simulink model "sampleModel653"  (R2023a)
settings: Solver=VariableStepAuto  StartTime=0.0  StopTime=10.0  RelTol=1e-3
undefined symbols (not defined in the file): DiscIntNeverNeededParam, magnitude, Newton, Raphson
libraries: simulink x238, slpidlib x68
(part 3 of 11)

== system sampleModel653/cfblk161 ==
  cfblk1 : Inport
  cfblk15 : Inport  Port=2
  cfblk10 : Product  Inputs=*
  cfblk11 : Signum
  cfblk12 : Constant  Value=[-980980330.453892]  SampleTime=1
  cfblk13 : Subsystem
  cfblk14 : Subsystem
  cfblk3 : DiscreteFir  SampleTime=1
  cfblk4 : slpidlib/PID Controller  Controller=PID  Form=Parallel  TimeDomain=Discrete-time  UseExternalTs=off  SampleTime=1  IntegratorMethod=Forward Euler  FilterMethod=Forward Euler  ControllerParametersSource=internal  P=1  I=1  UseKiTs=off  D=0  N=100  UseFilter=on  TunerSelectOption=Transfer Function Based (PID Tuner App)  InitialConditionSource=internal  InitialConditionForIntegrator=0  InitialConditionForFilter=0  DifferentiatorICPrevScaledInput=0  ExternalReset=none  TrackingMode=off  Kt=1  LimitOutput=off  SatLimitsSource=internal  UpperSaturationLimit=inf  LowerSaturationLimit=-inf  LinearizeAsGain=off  AntiWindupMode=none  Kb=1  LimitIntegrator=off  UpperIntegratorSaturationLimit=inf  LowerIntegratorSaturationLimit=-inf  POutMin=[]  POutMax=[]  IOutMin=[]  IOutMax=[]  DOutMin=[]  DOutMax=[]  NOutMin=[]  NOutMax=[]  SumOutMin=[]  SumOutMax=[]  SaturationOutMin=[]  SaturationOutMax=[]  PParamMin=[]  PParamMax=[]  IParamMin=[]  IParamMax=[]  DParamMin=[]  DParamMax=[]  NParamMin=[]  NParamMax=[]  KbParamMin=[]  KbParamMax=[]  KtParamMin=[]  KtParamMax=[]  KbOutMin=[]  KbOutMax=[]  KtOutMin=[]  KtOutMax=[]  IntegratorOutMin=[]  IntegratorOutMax=[]  FilterOutMin=[]  FilterOutMax=[]  SumI1OutMin=[]  SumI1OutMax=[]  SumI2OutMin=[]  SumI2OutMax=[]  SumI3OutMin=[]  SumI3OutMax=[]  SumI4OutMin=[]  SumI4OutMax=[]  SumDOutMin=[]  SumDOutMax=[]  DifferentiatorOutMin=[]  DifferentiatorOutMax=[]  FilterDiffOutCoefMin=[]  FilterDiffOutCoefMax=[]  ReciprocalOutMin=[]  ReciprocalOutMax=[]  SumDenOutMin=[]  SumDenOutMax=[]  SumNumOutMin=[]  SumNumOutMax=[]  DivideOutMin=[]  DivideOutMax=[]  UdiffTsProdOutMin=[]  UdiffTsProdOutMax=[]  NTsProdOutMin=[]  NTsProdOutMax=[]  UintegralTsProdOutMin=[]  UintegralTsProdOutMax=[]  UngainTsProdOutMin=[]  UngainTsProdOutMax=[]  ClampingZeroOutDataTypeStr=Inherit: Inherit via back propagation  ClampingZeroOutMin=[]  ClampingZeroOutMax=[]  FilterDenConstantOutDataTypeStr=Inherit: Inherit via back propagation  FilterDenConstantOutMin=[]  FilterDenConstantOutMax=[]  PCopyOutDataTypeStr=Inherit: Inherit via back propagation  PCopyOutMin=[]  PCopyOutMax=[]  NCopyOutDataTypeStr=Inherit: Inherit via back propagation  NCopyOutMin=[]  NCopyOutMax=[]  IntegratorContinuousStateAttributes=''  IntegratorStateMustResolveToSignalObject=off  IntegratorRTWStateStorageClass=Auto  FilterContinuousStateAttributes=''  FilterStateMustResolveToSignalObject=off  FilterRTWStateStorageClass=Auto  ParallelPVariant=InternalParameters  IdealPVariant=Disabled  IVariant=InternalParameters  DVariant=InternalParameters  IntegratorVariant=Discrete  SatVariant=Disabled  AWVariant=Passthrough  PCopyVariant=Disabled  TRVariant=Disabled  FdbkBlocksVariant=Forward  IdealPFdbkVariant=Disabled  SatFdbkVariant=Disabled  DerivativeFilterVariant=ForwardEulerFilter  NVariant=InternalParameters  NCopyVariant=Disabled  FilterICVariant=InternalICsFilter  IntegratorICVariant=InternalICs  ExternalResetVariant=Disabled  TRSumVariant=Passthrough  SumFdbkVariant=Disabled  SumVariant=Sum_PID  TsampFilterVariant=InternalTs  TsampNgainVariant=Passthrough  TsampIntegralVariant=Disabled_SignalSpec  ExternalSaturationOutDataTypeStr=Inherit: Same as second input
      settings: LibrarySourceBlock=simulink/Discrete/Discrete PID Controller
  cfblk5 : simulink/Discrete/Tapped Delay  vinit=0.0  samptime=-1  NumDelays=1  DelayOrder=Oldest  includeCurrent=off
  cfblk6 : Sum  Inputs=+-
  cfblk7 : Sqrt  Operator=rSqrt  AlgorithmType=Newton-Raphson
  cfblk8 : ComplexToMagnitudeAngle
  cfblk9 : Math  Operator=conj
  cfblk2 : Outport
  cfblk16 : Outport  Port=2
  wires:
  cfblk7/1 -> cfblk6/1
  cfblk14/1(cfblk2) -> cfblk16/1
  cfblk4/1 -> cfblk7/1
  cfblk6/1 -> cfblk14/1(cfblk1)
  cfblk12/1 -> cfblk8/1
  cfblk5/1 -> cfblk3/1
  cfblk9/1 -> cfblk14/2(cfblk6)
  cfblk14/2(cfblk7) -> cfblk10/1
  cfblk8/1 -> cfblk13/1(cfblk1)
  cfblk11/1 -> cfblk9/1
  cfblk15/1 -> cfblk13/2(cfblk13)
  cfblk13/1(cfblk2) -> cfblk6/2
  cfblk3/1 -> cfblk11/1
  cfblk8/2 -> cfblk5/1
  cfblk1/1 -> cfblk4/1
  cfblk13/2(cfblk14) -> cfblk2/1

== system sampleModel653/cfblk162 ==
  cfblk1 : Inport
  cfblk12 : Inport  Port=2
  cfblk13 : Inport  Port=3
  cfblk10 : Subsystem
  cfblk11 : Subsystem
  cfblk{14..17} (4 alike) : Delay  SampleTime=1
  cfblk3 : DiscreteStateSpace
  cfblk4 : simulink/Discrete/Difference  ICPrevInput=0.0  OutMin=[]  OutMax=[]  OutDataTypeStr=Inherit: Inherit via back propagation  OutDataType=fixdt(1, 16)  OutScaling=2^-10  DoSatur=off
  cfblk5 : simulink/Math Operations/Slider Gain  gain=1  low=0  high=2
  cfblk6 : Constant  Value=[520175118.847809]  SampleTime=1
  cfblk7 : Subsystem
  cfblk8 : Subsystem
  cfblk9 : Subsystem
  cfblk2 : Outport
  wires:
  cfblk7/1(cfblk2) -> cfblk4/1
  cfblk12/1 -> cfblk11/1(cfblk1)
  cfblk11/1(cfblk2) -> cfblk3/1
  cfblk13/1 -> cfblk7/1(cfblk1)
  cfblk6/1 -> cfblk11/3(cfblk15), cfblk10/2(cfblk6)
  cfblk1/1 -> cfblk11/4(cfblk16)
  cfblk5/1 -> cfblk8/2(cfblk7)
  cfblk7/2(cfblk15) -> cfblk5/1
  cfblk8/2(cfblk9) -> cfblk9/1(cfblk1)
  cfblk10/1(cfblk2) -> cfblk2/1
  cfblk8/3(cfblk10) -> cfblk9/2(cfblk14)
  cfblk3/1 -> cfblk7/3(cfblk14)
  cfblk7/3(cfblk16) -> cfblk9/3(cfblk15)
  cfblk9/3(cfblk17) -> cfblk10/1(cfblk1)
  cfblk4/1 -> cfblk14/1
  cfblk14/1 -> cfblk11/2(cfblk14)
  cfblk8/1(cfblk2) -> cfblk15/1
  cfblk15/1 -> cfblk7/2(cfblk13)
  cfblk9/1(cfblk2) -> cfblk16/1
  cfblk16/1 -> cfblk8/1(cfblk1)
  cfblk9/2(cfblk16) -> cfblk17/1
  cfblk17/1 -> cfblk8/3(cfblk8)

== system sampleModel653/cfblk163 ==
  cfblk1 : Inport
  cfblk3 : simulink/Discrete/Transfer Fcn First Order  PoleZ=0.95  ICPrevOutput=0.0  DoSatur=off
  cfblk4 : Product  Inputs=**
  cfblk5 : Sum  Inputs=--
  cfblk6 : Abs  SaturateOnIntegerOverflow=off
  cfblk7 : Constant  Value=[266211671.237557]  SampleTime=1
  cfblk2 : Outport
  cfblk8 : Outport  Port=2
  cfblk9 : Outport  Port=3
  wires:
  cfblk1/1 -> cfblk6/1
  cfblk3/1 -> cfblk5/1
  cfblk4/1 -> cfblk9/1
  cfblk6/1 -> cfblk5/2, cfblk3/1
  cfblk5/1 -> cfblk4/1, cfblk8/1
  cfblk7/1 -> cfblk2/1, cfblk4/2

== system sampleModel653/cfblk164 ==
  cfblk1 : Inport
  cfblk7 : Inport  Port=2
  cfblk8 : Inport  Port=3
  cfblk3 : simulink/Discrete/Transfer Fcn First Order  PoleZ=0.95  ICPrevOutput=0.0  DoSatur=off
  cfblk4 : simulink/Discrete/Transfer Fcn Real Zero  ZeroZ=0.75  ICPrevInput=0.0  DoSatur=off
  cfblk5 : Constant  Value=[908519091.701283]  SampleTime=1
  cfblk6 : Subsystem
  cfblk9 : Delay  SampleTime=1
  cfblk2 : Outport
  wires:
  cfblk1/1 -> cfblk2/1, cfblk6/5(cfblk15)
  cfblk5/1 -> cfblk6/1(cfblk1)
  cfblk4/1 -> cfblk6/2(cfblk12)
  cfblk6/1(cfblk2) -> cfblk3/1
  cfblk8/1 -> cfblk6/4(cfblk14)
  cfblk7/1 -> cfblk4/1
  cfblk3/1 -> cfblk9/1
  cfblk9/1 -> cfblk6/3(cfblk13)

== system sampleModel653/cfblk165 ==
  cfblk1 : Inport
  cfblk8 : Inport  Port=2
  cfblk9 : Inport  Port=3
  cfblk3 : simulink/Discrete/Tapped Delay  vinit=0.0  samptime=-1  NumDelays=1  DelayOrder=Oldest  includeCurrent=off
  cfblk4 : UnitDelay  HasFrameUpgradeWarning=on
  cfblk5 : Sqrt
  cfblk6 : ComplexToMagnitudeAngle
  cfblk7 : Subsystem
  cfblk2 : Outport
  cfblk10 : Outport  Port=2
  wires:
  cfblk4/1 -> cfblk10/1
  cfblk5/1 -> cfblk7/1(cfblk1)
  cfblk3/1 -> cfblk6/1
  cfblk6/1 -> cfblk4/1
  cfblk7/1(cfblk2) -> cfblk3/1
  cfblk1/1 -> cfblk5/1
  cfblk7/2(cfblk6) -> cfblk2/1

== system sampleModel653/cfblk166 ==
  cfblk1 : Inport
  cfblk{4,11..15} (6 alike) : Delay  SampleTime=1
  cfblk3 : Delay  DelayLengthSource=Input port  SampleTime=1
      settings: InputPortMap=u0,p1
  cfblk5 : Sqrt  Operator=rSqrt  AlgorithmType=Newton-Raphson
  cfblk6 : Product  Inputs=*
  cfblk7 : Subsystem
  cfblk2 : Outport
  cfblk8 : Outport  Port=2
  cfblk9 : Outport  Port=3
  cfblk10 : Outport  Port=4
  wires:
  cfblk4/1 -> cfblk8/1, cfblk12/1, cfblk13/1
  cfblk3/1 -> cfblk4/1, cfblk2/1, cfblk11/1, cfblk14/1
  cfblk1/1 -> cfblk6/1, cfblk7/5(cfblk13), cfblk7/6(cfblk14)
  cfblk7/1(cfblk2) -> cfblk5/1, cfblk9/1
  cfblk6/1 -> cfblk10/1, cfblk7/3(cfblk11)
  cfblk5/1 -> cfblk3/2, cfblk15/1
  cfblk11/1 -> cfblk7/1(cfblk1)
  cfblk12/1 -> cfblk3/1
  cfblk13/1 -> cfblk7/4(cfblk12)
  cfblk14/1 -> cfblk7/2(cfblk10)
  cfblk15/1 -> cfblk7/7(cfblk15)

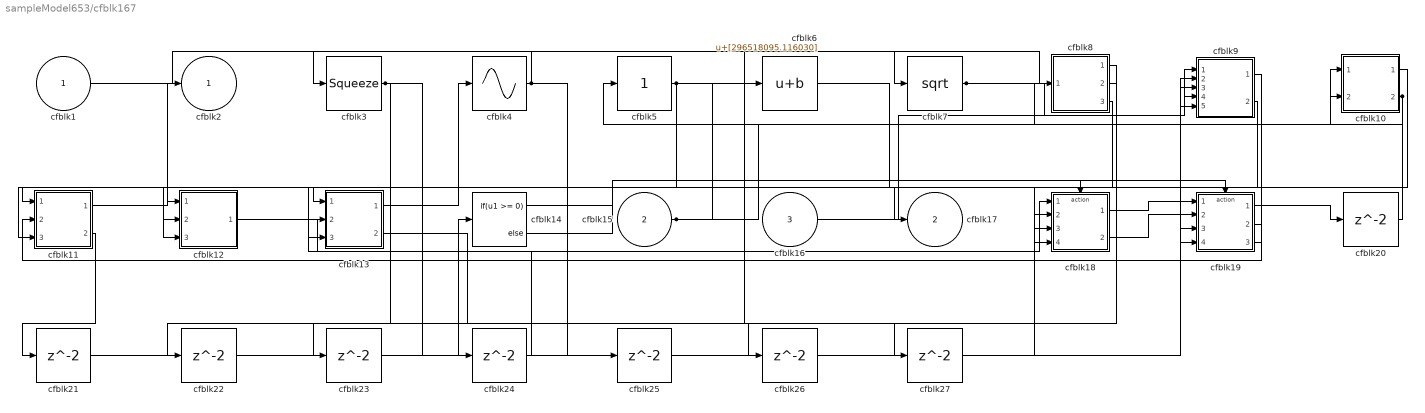
== system sampleModel653/cfblk167 ==
  cfblk1 : Inport
  cfblk15 : Inport  Port=2
  cfblk16 : Inport  Port=3
  cfblk10 : Subsystem
  cfblk11 : Subsystem
  cfblk12 : Subsystem
  cfblk13 : Subsystem
  cfblk14 : If  IfExpression=u1 >= 0  SampleTime=1
  cfblk18 : Subsystem  TreatAsAtomicUnit=on
  cfblk19 : Subsystem  TreatAsAtomicUnit=on
  cfblk{20..27} (8 alike) : Delay  SampleTime=1
  cfblk3 : Squeeze
  cfblk4 : Sin  TimeSource=Use external signal  SampleTime=0
  cfblk5 : simulink/Math Operations/Slider Gain  gain=1  low=0  high=2
  cfblk6 : Bias  Bias=[296518095.116030]  SaturateOnIntegerOverflow=off
  cfblk7 : Sqrt
  cfblk8 : Subsystem
  cfblk9 : Subsystem
  cfblk2 : Outport
  cfblk17 : Outport  Port=2
  wires:
  cfblk16/1 -> cfblk9/1(cfblk1)
  cfblk5/1 -> cfblk11/1(cfblk1), cfblk8/1(cfblk1), cfblk13/3(cfblk16), cfblk27/1
  cfblk13/1(cfblk2) -> cfblk4/1
  cfblk12/1(cfblk2) -> cfblk18/1(cfblk1)
  cfblk15/1 -> cfblk6/1, cfblk10/1(cfblk1)
  cfblk1/1 -> cfblk7/1
  cfblk11/1(cfblk2) -> cfblk2/1
  cfblk9/1(cfblk2) -> cfblk12/1(cfblk1)
  cfblk19/2(cfblk16) -> cfblk11/2(cfblk14)
  cfblk4/1 -> cfblk3/1, cfblk25/1
  cfblk19/3(cfblk17) -> cfblk5/1
  cfblk3/1 -> cfblk23/1, cfblk24/1
  cfblk6/1 -> cfblk18/4(cfblk12)
  cfblk9/2(cfblk15) -> cfblk12/2(cfblk10)
  cfblk10/1(cfblk2) -> cfblk13/1(cfblk1)
  cfblk8/1(cfblk2) -> cfblk17/1
  cfblk10/2(cfblk10) -> cfblk12/3(cfblk11), cfblk19/4(cfblk15)
  cfblk18/1(cfblk2) -> cfblk19/1(cfblk1)
  cfblk18/2(cfblk13) -> cfblk19/2(cfblk13)
  cfblk7/1 -> cfblk9/4(cfblk13), cfblk10/2(cfblk9)
  cfblk8/3(cfblk8) -> cfblk11/3(cfblk15)
  cfblk14/1 -> cfblk18/Action
  cfblk14/2 -> cfblk19/Action
  cfblk19/1(cfblk2) -> cfblk20/1
  cfblk20/1 -> cfblk9/2(cfblk11)
  cfblk11/2(cfblk16) -> cfblk21/1
  cfblk21/1 -> cfblk18/3(cfblk11)
  cfblk8/2(cfblk7) -> cfblk22/1
  cfblk22/1 -> cfblk14/1
  cfblk23/1 -> cfblk9/3(cfblk12)
  cfblk24/1 -> cfblk13/2(cfblk15)
  cfblk25/1 -> cfblk19/3(cfblk14)
  cfblk13/2(cfblk17) -> cfblk26/1
  cfblk26/1 -> cfblk18/2(cfblk10)
  cfblk27/1 -> cfblk9/5(cfblk14)

== system sampleModel653/cfblk168 ==
  cfblk1 : Inport
  cfblk10 : Inport  Port=2
  cfblk11 : Inport  Port=3
  cfblk13 : Delay  SampleTime=1
  cfblk3 : DiscreteStateSpace
  cfblk4 : DiscreteZeroPole  Poles=[0 0.5]  Gain=1
  cfblk5 : Rounding
  cfblk6 : Constant  Value=[-270536108.495275]  SampleTime=1
  cfblk7 : Subsystem
  cfblk8 : Subsystem
  cfblk9 : Subsystem
  cfblk2 : Outport
  cfblk12 : Outport  Port=2
  wires:
  cfblk1/1 -> cfblk7/1(cfblk1)
  cfblk11/1 -> cfblk8/1(cfblk1)
  cfblk6/1 -> cfblk8/2(cfblk10)
  cfblk3/1 -> cfblk2/1
  cfblk9/1(cfblk2) -> cfblk12/1
  cfblk4/1 -> cfblk9/1(cfblk1)
  cfblk8/1(cfblk2) -> cfblk3/1
  cfblk10/1 -> cfblk5/1
  cfblk8/2(cfblk11) -> cfblk9/2(cfblk8)
  cfblk9/2(cfblk9) -> cfblk13/1
  cfblk13/1 -> cfblk4/1

== system sampleModel653/cfblk169 ==
  cfblk1 : Inport
  cfblk7 : Inport  Port=2
  cfblk3 : Constant  Value=[373927512.445673]  SampleTime=1
  cfblk4 : Constant  Value=[-436487022.604392]  SampleTime=1
  cfblk5 : Subsystem
  cfblk6 : Subsystem
  cfblk8 : Delay  SampleTime=1
  cfblk2 : Outport
  wires:
  cfblk1/1 -> cfblk2/1
  cfblk6/1(cfblk2) -> cfblk5/1(cfblk1)
  cfblk7/1 -> cfblk6/1(cfblk1)
  cfblk4/1 -> cfblk6/3(cfblk10)
  cfblk5/1(cfblk2) -> cfblk8/1
  cfblk8/1 -> cfblk6/2(cfblk9)

== system sampleModel653/cfblk170 ==
  cfblk1 : Inport
  cfblk13 : Inport  Port=2
  cfblk14 : Inport  Port=3
  cfblk10 : Subsystem
  cfblk11 : Subsystem
  cfblk12 : Subsystem
  cfblk15 : Delay  SampleTime=1
  cfblk16 : Delay  SampleTime=1
  cfblk3 : Sum  Inputs=+-
  cfblk4 : UnaryMinus
  cfblk5 : Sum  Inputs=+-
  cfblk6 : Rounding
  cfblk7 : simulink/Math Operations/Slider Gain  gain=1  low=0  high=2
  cfblk8 : Sum  Inputs=+-
  cfblk9 : Constant  Value=[279332915.374205]  SampleTime=1
  cfblk2 : Outport
  wires:
  cfblk13/1 -> cfblk6/1, cfblk10/4(cfblk15)
  cfblk1/1 -> cfblk3/1
  cfblk6/1 -> cfblk7/1, cfblk10/3(cfblk14)
  cfblk9/1 -> cfblk10/1(cfblk1), cfblk11/3(cfblk15)
  cfblk11/1(cfblk2) -> cfblk5/1
  cfblk4/1 -> cfblk11/1(cfblk1), cfblk11/4(cfblk16)
  cfblk14/1 -> cfblk5/2
  cfblk7/1 -> cfblk4/1
  cfblk10/1(cfblk2) -> cfblk12/1(cfblk1)
  cfblk12/1(cfblk2) -> cfblk8/1
  cfblk5/1 -> cfblk8/2
  cfblk11/2(cfblk17) -> cfblk2/1
  cfblk3/1 -> cfblk11/2(cfblk14)
  cfblk8/1 -> cfblk15/1
  cfblk15/1 -> cfblk3/2
  cfblk12/2(cfblk8) -> cfblk16/1
  cfblk16/1 -> cfblk10/2(cfblk13)

== system sampleModel653/cfblk171 ==
  cfblk1 : Inport
  cfblk8 : Inport  Port=2
  cfblk9 : Inport  Port=3
  cfblk11 : Delay  SampleTime=1
  cfblk3 : slpidlib/PID Controller (2DOF)  Controller=PID  Form=Parallel  TimeDomain=Discrete-time  UseExternalTs=off  SampleTime=1  IntegratorMethod=Forward Euler  FilterMethod=Forward Euler  ControllerParametersSource=internal  P=1  I=1  UseKiTs=off  D=0  N=100  UseFilter=on  b=1  c=1  TunerSelectOption=Transfer Function Based (PID Tuner App)  InitialConditionSource=internal  InitialConditionForIntegrator=0  InitialConditionForFilter=0  DifferentiatorICPrevScaledInput=0  ExternalReset=none  TrackingMode=off  Kt=1  LimitOutput=off  SatLimitsSource=internal  UpperSaturationLimit=inf  LowerSaturationLimit=-inf  LinearizeAsGain=off  AntiWindupMode=none  Kb=1  LimitIntegrator=off  UpperIntegratorSaturationLimit=inf  LowerIntegratorSaturationLimit=-inf  POutMin=[]  POutMax=[]  IOutMin=[]  IOutMax=[]  DOutMin=[]  DOutMax=[]  NOutMin=[]  NOutMax=[]  bOutMin=[]  bOutMax=[]  cOutMin=[]  cOutMax=[]  SumOutMin=[]  SumOutMax=[]  SaturationOutMin=[]  SaturationOutMax=[]  PParamMin=[]  PParamMax=[]  IParamMin=[]  IParamMax=[]  DParamMin=[]  DParamMax=[]  NParamMin=[]  NParamMax=[]  bParamMin=[]  bParamMax=[]  cParamMin=[]  cParamMax=[]  KbParamMin=[]  KbParamMax=[]  KtParamMin=[]  KtParamMax=[]  KbOutMin=[]  KbOutMax=[]  KtOutMin=[]  KtOutMax=[]  IntegratorOutMin=[]  IntegratorOutMax=[]  FilterOutMin=[]  FilterOutMax=[]  SumI1OutMin=[]  SumI1OutMax=[]  SumI2OutMin=[]  SumI2OutMax=[]  SumI3OutMin=[]  SumI3OutMax=[]  SumI4OutMin=[]  SumI4OutMax=[]  SumDOutMin=[]  SumDOutMax=[]  Sum1OutMin=[]  Sum1OutMax=[]  Sum2OutMin=[]  Sum2OutMax=[]  Sum3OutMin=[]  Sum3OutMax=[]  DifferentiatorOutMin=[]  DifferentiatorOutMax=[]  FilterDiffOutCoefMin=[]  FilterDiffOutCoefMax=[]  ReciprocalOutMin=[]  ReciprocalOutMax=[]  SumDenOutMin=[]  SumDenOutMax=[]  SumNumOutMin=[]  SumNumOutMax=[]  DivideOutMin=[]  DivideOutMax=[]  UdiffTsProdOutMin=[]  UdiffTsProdOutMax=[]  NTsProdOutMin=[]  NTsProdOutMax=[]  UintegralTsProdOutMin=[]  UintegralTsProdOutMax=[]  UngainTsProdOutMin=[]  UngainTsProdOutMax=[]  ClampingZeroOutDataTypeStr=Inherit: Inherit via back propagation  ClampingZeroOutMin=[]  ClampingZeroOutMax=[]  FilterDenConstantOutDataTypeStr=Inherit: Inherit via back propagation  FilterDenConstantOutMin=[]  FilterDenConstantOutMax=[]  PCopyOutDataTypeStr=Inherit: Inherit via back propagation  PCopyOutMin=[]  PCopyOutMax=[]  NCopyOutDataTypeStr=Inherit: Inherit via back propagation  NCopyOutMin=[]  NCopyOutMax=[]  IntegratorContinuousStateAttributes=''  IntegratorStateMustResolveToSignalObject=off  IntegratorRTWStateStorageClass=Auto  FilterContinuousStateAttributes=''  FilterStateMustResolveToSignalObject=off  FilterRTWStateStorageClass=Auto  ParallelPVariant=InternalParameters  IdealPVariant=Disabled  IVariant=InternalParameters  DVariant=InternalParameters  bVariant=InternalParameters  cVariant=InternalParameters  IntegratorVariant=Discrete  SatVariant=Disabled  AWVariant=Passthrough  PCopyVariant=Disabled  TRVariant=Disabled  FdbkBlocksVariant=Forward  IdealPFdbkVariant=Disabled  SatFdbkVariant=Disabled  DerivativeFilterVariant=ForwardEulerFilter  NVariant=InternalParameters  NCopyVariant=Disabled  FilterICVariant=InternalICsFilter  IntegratorICVariant=InternalICs  ExternalResetVariant=Disabled  TRSumVariant=Passthrough  SumFdbkVariant=Disabled  SumVariant=Sum_PID  TsampFilterVariant=InternalTs  TsampNgainVariant=Passthrough  TsampIntegralVariant=Disabled_SignalSpec  ExternalSaturationOutDataTypeStr=Inherit: Same as second input
      settings: LibrarySourceBlock=simulink/Discrete/Discrete PID Controller (2DOF)
  cfblk4 : Gain  Gain=[-457446233.510132]
  cfblk5 : Constant  Value=[-436711553.418226]  SampleTime=1
  cfblk6 : Subsystem
  cfblk7 : Subsystem
  cfblk2 : Outport
  cfblk10 : Outport  Port=2
  wires:
  cfblk7/1(cfblk2) -> cfblk10/1
  cfblk5/1 -> cfblk2/1
  cfblk4/1 -> cfblk6/1(cfblk1), cfblk7/3(cfblk7)
  cfblk1/1 -> cfblk7/1(cfblk1)
  cfblk8/1 -> cfblk6/2(cfblk15), cfblk3/2
  cfblk9/1 -> cfblk6/3(cfblk16)
  cfblk6/1(cfblk2) -> cfblk7/2(cfblk6), cfblk11/1
  cfblk3/1 -> cfblk4/1
  cfblk11/1 -> cfblk3/1

== system sampleModel653/cfblk172 ==
  cfblk1 : Inport
  cfblk6 : Inport  Port=2
  cfblk{10..13} (4 alike) : Delay  SampleTime=1
  cfblk3 : Delay  ShowEnablePort=on  SampleTime=1
      settings: InputPortMap=u0,e6
  cfblk4 : Sum  Inputs=--
  cfblk5 : Subsystem
  cfblk2 : Outport
  cfblk7 : Outport  Port=2
  cfblk8 : Outport  Port=3
  cfblk9 : Outport  Port=4
  wires:
  cfblk4/1 -> cfblk8/1, cfblk5/5(cfblk12)
  cfblk6/1 -> cfblk3/1, cfblk9/1
  cfblk5/1(cfblk2) -> cfblk3/2
  cfblk1/1 -> cfblk4/2, cfblk5/2(cfblk9)
  cfblk3/1 -> cfblk2/1, cfblk7/1, cfblk10/1, cfblk11/1, cfblk12/1
  cfblk10/1 -> cfblk5/1(cfblk1)
  cfblk11/1 -> cfblk5/3(cfblk10)
  cfblk12/1 -> cfblk5/4(cfblk11)
  cfblk5/2(cfblk13) -> cfblk13/1
  cfblk13/1 -> cfblk4/1

== system sampleModel653/cfblk173 ==
  cfblk1 : Inport
  cfblk7 : Inport  Port=2
  cfblk3 : Delay  DelayLengthSource=Input port  SampleTime=1
      settings: InputPortMap=u0,p1
  cfblk4 : DiscreteZeroPole  Poles=[0 0.5]  Gain=1
  cfblk5 : Signum
  cfblk6 : Subsystem
  cfblk8 : Delay  SampleTime=1
  cfblk2 : Outport
  wires:
  cfblk6/1(cfblk2) -> cfblk4/1
  cfblk4/1 -> cfblk2/1
  cfblk6/2(cfblk9) -> cfblk3/1
  cfblk5/1 -> cfblk3/2
  cfblk7/1 -> cfblk5/1
  cfblk1/1 -> cfblk6/1(cfblk1)
  cfblk3/1 -> cfblk8/1
  cfblk8/1 -> cfblk6/2(cfblk8)

== system sampleModel653/cfblk183 ==
  cfblk1 : Inport
  cfblk8 : Inport  Port=2
  Action Port : ActionPort  ActionPortLabel=if(u1 >= 0)
  cfblk3 : Squeeze
  cfblk4 : Reshape
  cfblk5 : Constant  Value=[-334139740.220997]  SampleTime=1
  cfblk6 : Constant  Value=[-428556013.443740]  SampleTime=1
  cfblk7 : Subsystem
  cfblk2 : Outport
  wires:
  cfblk5/1 -> cfblk2/1
  cfblk6/1 -> cfblk4/1
  cfblk1/1 -> cfblk3/1
  cfblk4/1 -> cfblk7/1(cfblk1)
  cfblk8/1 -> cfblk7/2(cfblk15)
  cfblk3/1 -> cfblk7/3(cfblk16)

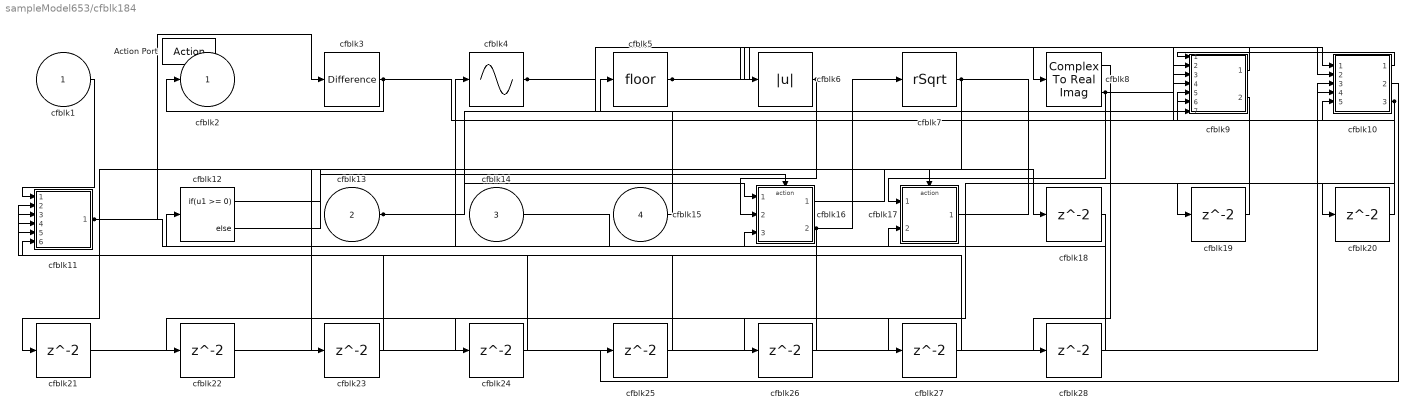
== system sampleModel653/cfblk184 ==
  cfblk1 : Inport
  cfblk13 : Inport  Port=2
  cfblk14 : Inport  Port=3
  cfblk15 : Inport  Port=4
  Action Port : ActionPort  ActionPortLabel=else
  cfblk10 : Subsystem
  cfblk11 : Subsystem
  cfblk12 : If  IfExpression=u1 >= 0  SampleTime=1
  cfblk16 : Subsystem  TreatAsAtomicUnit=on
  cfblk17 : Subsystem  TreatAsAtomicUnit=on
  cfblk{18..28} (11 alike) : Delay
  cfblk3 : simulink/Discrete/Difference  ICPrevInput=0.0  OutMin=[]  OutMax=[]  OutDataTypeStr=Inherit: Inherit via back propagation  OutDataType=fixdt(1, 16)  OutScaling=2^-10  DoSatur=off
  cfblk4 : Sin  TimeSource=Use external signal  SampleTime=0
  cfblk5 : Rounding
  cfblk6 : Abs  SaturateOnIntegerOverflow=off
  cfblk7 : Sqrt  Operator=rSqrt  AlgorithmType=Newton-Raphson
  cfblk8 : ComplexToRealImag
  cfblk9 : Subsystem
  cfblk2 : Outport
  wires:
  cfblk13/1 -> cfblk16/1(cfblk1), cfblk9/5(cfblk13)
  cfblk10/1(cfblk2) -> cfblk9/1(cfblk1)
  cfblk3/1 -> cfblk2/1, cfblk10/5(cfblk14)
  cfblk16/2(cfblk16) -> cfblk7/1, cfblk22/1
  cfblk6/1 -> cfblk16/2(cfblk14), cfblk23/1
  cfblk14/1 -> cfblk16/3(cfblk15)
  cfblk5/1 -> cfblk9/3(cfblk11), cfblk10/1(cfblk1)
  cfblk15/1 -> cfblk5/1
  cfblk11/1(cfblk2) -> cfblk3/1, cfblk17/2(cfblk8)
  cfblk9/1(cfblk2) -> cfblk6/1
  cfblk4/1 -> cfblk8/1, cfblk9/6(cfblk14)
  cfblk1/1 -> cfblk11/1(cfblk1)
  cfblk7/1 -> cfblk20/1, cfblk21/1
  cfblk8/2 -> cfblk17/1(cfblk1), cfblk10/2(cfblk11)
  cfblk10/3(cfblk16) -> cfblk9/7(cfblk15), cfblk26/1, cfblk27/1
  cfblk12/1 -> cfblk16/Action
  cfblk12/2 -> cfblk17/Action
  cfblk16/1(cfblk2) -> cfblk18/1
  cfblk18/1 -> cfblk12/1
  cfblk17/1(cfblk2) -> cfblk19/1
  cfblk19/1 -> cfblk9/2(cfblk10)
  cfblk20/1 -> cfblk9/4(cfblk12)
  cfblk21/1 -> cfblk10/3(cfblk12)
  cfblk22/1 -> cfblk10/4(cfblk13)
  cfblk23/1 -> cfblk11/5(cfblk14)
  cfblk9/2(cfblk16) -> cfblk24/1
  cfblk24/1 -> cfblk11/2(cfblk11)
  cfblk10/2(cfblk15) -> cfblk25/1
  cfblk25/1 -> cfblk11/3(cfblk12)
  cfblk26/1 -> cfblk11/4(cfblk13)
  cfblk27/1 -> cfblk11/6(cfblk15)
  cfblk8/1 -> cfblk28/1
  cfblk28/1 -> cfblk4/1

== system sampleModel653/cfblk185 ==
  cfblk1 : Inport
  Action Port : ActionPort  ActionPortLabel=if(u1 >= 0)
  cfblk10 : Constant  Value=[724663783.826056]  SampleTime=1
  cfblk11 : Subsystem
  cfblk12 : Subsystem
  cfblk3 : simulink/Discrete/Transfer Fcn First Order  PoleZ=0.95  ICPrevOutput=0.0  DoSatur=off
  cfblk4 : slpidlib/PID Controller  Controller=PID  Form=Parallel  TimeDomain=Discrete-time  UseExternalTs=off  SampleTime=-1  IntegratorMethod=Forward Euler  FilterMethod=Forward Euler  ControllerParametersSource=internal  P=1  I=1  UseKiTs=off  D=0  N=100  UseFilter=on  TunerSelectOption=Transfer Function Based (PID Tuner App)  InitialConditionSource=internal  InitialConditionForIntegrator=0  InitialConditionForFilter=0  DifferentiatorICPrevScaledInput=0  ExternalReset=none  TrackingMode=off  Kt=1  LimitOutput=off  SatLimitsSource=internal  UpperSaturationLimit=inf  LowerSaturationLimit=-inf  LinearizeAsGain=off  AntiWindupMode=none  Kb=1  LimitIntegrator=off  UpperIntegratorSaturationLimit=inf  LowerIntegratorSaturationLimit=-inf  POutMin=[]  POutMax=[]  IOutMin=[]  IOutMax=[]  DOutMin=[]  DOutMax=[]  NOutMin=[]  NOutMax=[]  SumOutMin=[]  SumOutMax=[]  SaturationOutMin=[]  SaturationOutMax=[]  PParamMin=[]  PParamMax=[]  IParamMin=[]  IParamMax=[]  DParamMin=[]  DParamMax=[]  NParamMin=[]  NParamMax=[]  KbParamMin=[]  KbParamMax=[]  KtParamMin=[]  KtParamMax=[]  KbOutMin=[]  KbOutMax=[]  KtOutMin=[]  KtOutMax=[]  IntegratorOutMin=[]  IntegratorOutMax=[]  FilterOutMin=[]  FilterOutMax=[]  SumI1OutMin=[]  SumI1OutMax=[]  SumI2OutMin=[]  SumI2OutMax=[]  SumI3OutMin=[]  SumI3OutMax=[]  SumI4OutMin=[]  SumI4OutMax=[]  SumDOutMin=[]  SumDOutMax=[]  DifferentiatorOutMin=[]  DifferentiatorOutMax=[]  FilterDiffOutCoefMin=[]  FilterDiffOutCoefMax=[]  ReciprocalOutMin=[]  ReciprocalOutMax=[]  SumDenOutMin=[]  SumDenOutMax=[]  SumNumOutMin=[]  SumNumOutMax=[]  DivideOutMin=[]  DivideOutMax=[]  UdiffTsProdOutMin=[]  UdiffTsProdOutMax=[]  NTsProdOutMin=[]  NTsProdOutMax=[]  UintegralTsProdOutMin=[]  UintegralTsProdOutMax=[]  UngainTsProdOutMin=[]  UngainTsProdOutMax=[]  ClampingZeroOutDataTypeStr=Inherit: Inherit via back propagation  ClampingZeroOutMin=[]  ClampingZeroOutMax=[]  FilterDenConstantOutDataTypeStr=Inherit: Inherit via back propagation  FilterDenConstantOutMin=[]  FilterDenConstantOutMax=[]  PCopyOutDataTypeStr=Inherit: Inherit via back propagation  PCopyOutMin=[]  PCopyOutMax=[]  NCopyOutDataTypeStr=Inherit: Inherit via back propagation  NCopyOutMin=[]  NCopyOutMax=[]  IntegratorContinuousStateAttributes=''  IntegratorStateMustResolveToSignalObject=off  IntegratorRTWStateStorageClass=Auto  FilterContinuousStateAttributes=''  FilterStateMustResolveToSignalObject=off  FilterRTWStateStorageClass=Auto  ParallelPVariant=InternalParameters  IdealPVariant=Disabled  IVariant=InternalParameters  DVariant=InternalParameters  IntegratorVariant=Discrete  SatVariant=Disabled  AWVariant=Passthrough  PCopyVariant=Disabled  TRVariant=Disabled  FdbkBlocksVariant=Forward  IdealPFdbkVariant=Disabled  SatFdbkVariant=Disabled  DerivativeFilterVariant=ForwardEulerFilter  NVariant=InternalParameters  NCopyVariant=Disabled  FilterICVariant=InternalICsFilter  IntegratorICVariant=InternalICs  ExternalResetVariant=Disabled  TRSumVariant=Passthrough  SumFdbkVariant=Disabled  SumVariant=Sum_PID  TsampFilterVariant=InternalTs  TsampNgainVariant=Passthrough  TsampIntegralVariant=Disabled_SignalSpec  ExternalSaturationOutDataTypeStr=Inherit: Same as second input
      settings: LibrarySourceBlock=simulink/Discrete/Discrete PID Controller
  cfblk5 : DiscreteZeroPole  Poles=[0 0.5]  Gain=1  SampleTime=-1
  cfblk6 : ComplexToRealImag
  cfblk7 : UnaryMinus
  cfblk8 : simulink/Math Operations/MinMax Running Resettable  Function=min  vinit=0.0
  cfblk9 : Gain  Gain=[964015079.433562]
  cfblk2 : Outport
  cfblk13 : Outport  Port=2
  cfblk14 : Outport  Port=3
  wires:
  cfblk4/1 -> cfblk7/1
  cfblk7/1 -> cfblk13/1
  cfblk5/1 -> cfblk11/1(cfblk1)
  cfblk8/1 -> cfblk14/1
  cfblk1/1 -> cfblk9/1
  cfblk10/1 -> cfblk4/1
  cfblk9/1 -> cfblk12/1(cfblk1), cfblk5/1
  cfblk11/1(cfblk2) -> cfblk2/1
  cfblk12/1(cfblk2) -> cfblk8/1, cfblk6/1
  cfblk6/1 -> cfblk3/1
  cfblk3/1 -> cfblk8/2
  cfblk6/2 -> cfblk11/2(cfblk14)

== system sampleModel653/cfblk186 ==
  cfblk1 : Inport
  Action Port : ActionPort  ActionPortLabel=else
  cfblk10 : Subsystem
  cfblk11 : Subsystem
  cfblk12 : Delay
  cfblk3 : simulink/Discrete/Transfer Fcn Real Zero  ZeroZ=0.75  ICPrevInput=0.0  DoSatur=off
  cfblk4 : Delay
  cfblk5 : Product
  cfblk6 : Abs  SaturateOnIntegerOverflow=off
  cfblk7 : Sqrt  Operator=rSqrt  AlgorithmType=Newton-Raphson
  cfblk8 : Constant  Value=[-106947018.188129]  SampleTime=1
  cfblk9 : Constant  Value=[767459599.248018]  SampleTime=1
  cfblk2 : Outport
  wires:
  cfblk9/1 -> cfblk4/1
  cfblk3/1 -> cfblk2/1
  cfblk8/1 -> cfblk11/1(cfblk1)
  cfblk1/1 -> cfblk6/1
  cfblk4/1 -> cfblk7/1
  cfblk11/1(cfblk2) -> cfblk5/1
  cfblk6/1 -> cfblk10/2(cfblk10)
  cfblk10/1(cfblk2) -> cfblk11/2(cfblk7)
  cfblk10/2(cfblk11) -> cfblk3/1
  cfblk10/3(cfblk12) -> cfblk5/2
  cfblk5/1 -> cfblk12/1
  cfblk12/1 -> cfblk10/1(cfblk1)

== system sampleModel653/cfblk187 ==
  cfblk1 : Inport
  cfblk6 : Inport  Port=2
  Action Port : ActionPort  ActionPortLabel=if(u1 >= 0)
  cfblk3 : DiscreteTransferFcn
  cfblk4 : MinMax  Function=max  Inputs=2
  cfblk5 : Subsystem
  cfblk8 : Delay
  cfblk9 : Delay
  cfblk2 : Outport
  cfblk7 : Outport  Port=2
  wires:
  cfblk4/1 -> cfblk3/1
  cfblk6/1 -> cfblk2/1
  cfblk5/1(cfblk2) -> cfblk7/1
  cfblk5/2(cfblk9) -> cfblk4/1
  cfblk3/1 -> cfblk8/1, cfblk9/1
  cfblk1/1 -> cfblk5/1(cfblk1)
  cfblk8/1 -> cfblk4/2
  cfblk9/1 -> cfblk5/2(cfblk8)

== system sampleModel653/cfblk188 ==
  cfblk1 : Inport
  Action Port : ActionPort  ActionPortLabel=else
  cfblk10 : Subsystem
  cfblk11 : Subsystem
  cfblk12 : Subsystem
  cfblk{13..16} (4 alike) : Delay
  cfblk3 : DiscreteFir
  cfblk4 : Polyval  Coefs=[ +2.081618890e-019, -1.441693666e-014, +4.719686976e-010, -8.536869453e-006, +1.621573104e-001, -8.087801117e+001 ]
  cfblk5 : Constant  Value=[-528883414.455919]  SampleTime=1
  cfblk6 : Subsystem
  cfblk7 : Subsystem
  cfblk8 : Subsystem
  cfblk9 : Subsystem
  cfblk2 : Outport
  wires:
  cfblk3/1 -> cfblk11/1(cfblk1), cfblk6/2(cfblk9)
  cfblk11/1(cfblk2) -> cfblk7/1(cfblk1)
  cfblk12/1(cfblk2) -> cfblk8/1(cfblk1)
  cfblk12/2(cfblk16) -> cfblk6/1(cfblk1)
  cfblk1/1 -> cfblk10/1(cfblk1)
  cfblk9/1(cfblk2) -> cfblk4/1
  cfblk4/1 -> cfblk10/2(cfblk12)
  cfblk8/3(cfblk11) -> cfblk10/3(cfblk13), cfblk9/1(cfblk1), cfblk9/2(cfblk10)
  cfblk11/2(cfblk13) -> cfblk12/2(cfblk15)
  cfblk10/1(cfblk2) -> cfblk2/1
  cfblk5/1 -> cfblk7/2(cfblk10), cfblk6/3(cfblk10)
  cfblk6/1(cfblk2) -> cfblk8/3(cfblk8)
  cfblk6/2(cfblk11) -> cfblk8/4(cfblk9)
  cfblk6/3(cfblk12) -> cfblk7/3(cfblk11)
  cfblk7/1(cfblk2) -> cfblk13/1
  cfblk13/1 -> cfblk11/2(cfblk12)
  cfblk8/1(cfblk2) -> cfblk14/1
  cfblk14/1 -> cfblk3/1
  cfblk8/2(cfblk10) -> cfblk15/1
  cfblk15/1 -> cfblk12/1(cfblk1)
  cfblk9/2(cfblk11) -> cfblk16/1
  cfblk16/1 -> cfblk8/2(cfblk7)

== system sampleModel653/cfblk189 ==
  cfblk1 : Inport
  cfblk8 : Inport  Port=2
  cfblk9 : Inport  Port=3
  Action Port : ActionPort  ActionPortLabel=if(u1 >= 0)
  cfblk3 : simulink/Discrete/Tapped Delay  vinit=0.0  samptime=-1  NumDelays=1  DelayOrder=Oldest  includeCurrent=off
  cfblk4 : slpidlib/PID Controller (2DOF)  Controller=PID  Form=Parallel  TimeDomain=Discrete-time  UseExternalTs=off  SampleTime=-1  IntegratorMethod=Forward Euler  FilterMethod=Forward Euler  ControllerParametersSource=internal  P=1  I=1  UseKiTs=off  D=0  N=100  UseFilter=on  b=1  c=1  TunerSelectOption=Transfer Function Based (PID Tuner App)  InitialConditionSource=internal  InitialConditionForIntegrator=0  InitialConditionForFilter=0  DifferentiatorICPrevScaledInput=0  ExternalReset=none  TrackingMode=off  Kt=1  LimitOutput=off  SatLimitsSource=internal  UpperSaturationLimit=inf  LowerSaturationLimit=-inf  LinearizeAsGain=off  AntiWindupMode=none  Kb=1  LimitIntegrator=off  UpperIntegratorSaturationLimit=inf  LowerIntegratorSaturationLimit=-inf  POutMin=[]  POutMax=[]  IOutMin=[]  IOutMax=[]  DOutMin=[]  DOutMax=[]  NOutMin=[]  NOutMax=[]  bOutMin=[]  bOutMax=[]  cOutMin=[]  cOutMax=[]  SumOutMin=[]  SumOutMax=[]  SaturationOutMin=[]  SaturationOutMax=[]  PParamMin=[]  PParamMax=[]  IParamMin=[]  IParamMax=[]  DParamMin=[]  DParamMax=[]  NParamMin=[]  NParamMax=[]  bParamMin=[]  bParamMax=[]  cParamMin=[]  cParamMax=[]  KbParamMin=[]  KbParamMax=[]  KtParamMin=[]  KtParamMax=[]  KbOutMin=[]  KbOutMax=[]  KtOutMin=[]  KtOutMax=[]  IntegratorOutMin=[]  IntegratorOutMax=[]  FilterOutMin=[]  FilterOutMax=[]  SumI1OutMin=[]  SumI1OutMax=[]  SumI2OutMin=[]  SumI2OutMax=[]  SumI3OutMin=[]  SumI3OutMax=[]  SumI4OutMin=[]  SumI4OutMax=[]  SumDOutMin=[]  SumDOutMax=[]  Sum1OutMin=[]  Sum1OutMax=[]  Sum2OutMin=[]  Sum2OutMax=[]  Sum3OutMin=[]  Sum3OutMax=[]  DifferentiatorOutMin=[]  DifferentiatorOutMax=[]  FilterDiffOutCoefMin=[]  FilterDiffOutCoefMax=[]  ReciprocalOutMin=[]  ReciprocalOutMax=[]  SumDenOutMin=[]  SumDenOutMax=[]  SumNumOutMin=[]  SumNumOutMax=[]  DivideOutMin=[]  DivideOutMax=[]  UdiffTsProdOutMin=[]  UdiffTsProdOutMax=[]  NTsProdOutMin=[]  NTsProdOutMax=[]  UintegralTsProdOutMin=[]  UintegralTsProdOutMax=[]  UngainTsProdOutMin=[]  UngainTsProdOutMax=[]  ClampingZeroOutDataTypeStr=Inherit: Inherit via back propagation  ClampingZeroOutMin=[]  ClampingZeroOutMax=[]  FilterDenConstantOutDataTypeStr=Inherit: Inherit via back propagation  FilterDenConstantOutMin=[]  FilterDenConstantOutMax=[]  PCopyOutDataTypeStr=Inherit: Inherit via back propagation  PCopyOutMin=[]  PCopyOutMax=[]  NCopyOutDataTypeStr=Inherit: Inherit via back propagation  NCopyOutMin=[]  NCopyOutMax=[]  IntegratorContinuousStateAttributes=''  IntegratorStateMustResolveToSignalObject=off  IntegratorRTWStateStorageClass=Auto  FilterContinuousStateAttributes=''  FilterStateMustResolveToSignalObject=off  FilterRTWStateStorageClass=Auto  ParallelPVariant=InternalParameters  IdealPVariant=Disabled  IVariant=InternalParameters  DVariant=InternalParameters  bVariant=InternalParameters  cVariant=InternalParameters  IntegratorVariant=Discrete  SatVariant=Disabled  AWVariant=Passthrough  PCopyVariant=Disabled  TRVariant=Disabled  FdbkBlocksVariant=Forward  IdealPFdbkVariant=Disabled  SatFdbkVariant=Disabled  DerivativeFilterVariant=ForwardEulerFilter  NVariant=InternalParameters  NCopyVariant=Disabled  FilterICVariant=InternalICsFilter  IntegratorICVariant=InternalICs  ExternalResetVariant=Disabled  TRSumVariant=Passthrough  SumFdbkVariant=Disabled  SumVariant=Sum_PID  TsampFilterVariant=InternalTs  TsampNgainVariant=Passthrough  TsampIntegralVariant=Disabled_SignalSpec  ExternalSaturationOutDataTypeStr=Inherit: Same as second input
      settings: LibrarySourceBlock=simulink/Discrete/Discrete PID Controller (2DOF)
  cfblk5 : Delay
  cfblk6 : MinMax
  cfblk7 : Subsystem
  cfblk2 : Outport
  cfblk10 : Outport  Port=2
  wires:
  cfblk6/1 -> cfblk4/1, cfblk7/4(cfblk11)
  cfblk5/1 -> cfblk6/1, cfblk7/2(cfblk9)
  cfblk4/1 -> cfblk2/1
  cfblk9/1 -> cfblk5/1, cfblk7/3(cfblk10)
  cfblk3/1 -> cfblk4/2
  cfblk1/1 -> cfblk10/1, cfblk7/5(cfblk12)
  cfblk8/1 -> cfblk7/1(cfblk1)
  cfblk7/1(cfblk2) -> cfblk3/1

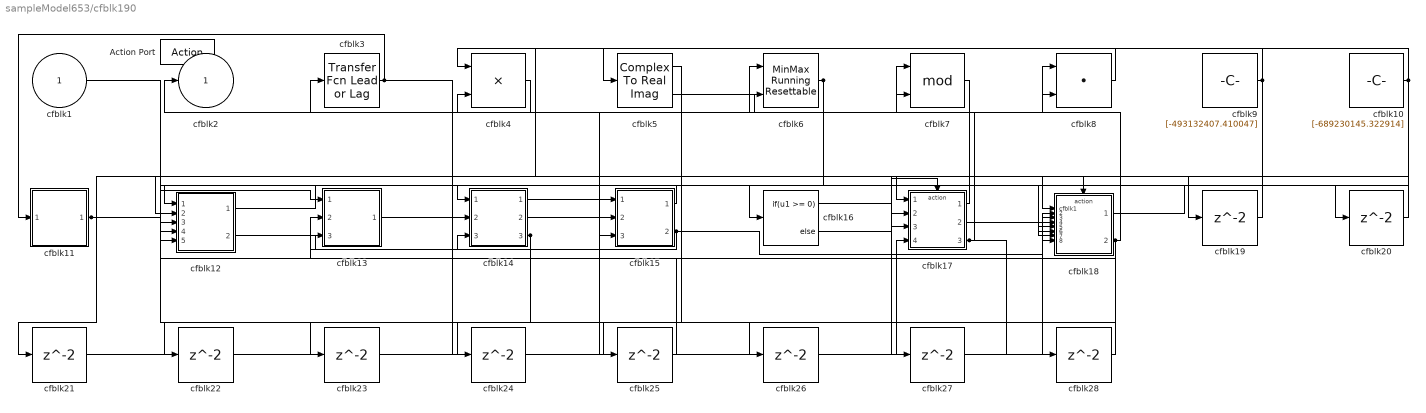
== system sampleModel653/cfblk190 ==
  cfblk1 : Inport
  Action Port : ActionPort  ActionPortLabel=else
  cfblk10 : Constant  Value=[-689230145.322914]  SampleTime=1
  cfblk11 : Subsystem
  cfblk12 : Subsystem
  cfblk13 : Subsystem
  cfblk14 : Subsystem
  cfblk15 : Subsystem
  cfblk16 : If  IfExpression=u1 >= 0  SampleTime=1
  cfblk17 : Subsystem  TreatAsAtomicUnit=on
  cfblk18 : Subsystem  TreatAsAtomicUnit=on
  cfblk{19..28} (10 alike) : Delay
  cfblk3 : simulink/Discrete/Transfer Fcn Lead or Lag  PoleZ=0.95  ZeroZ=0.75  ICPrevOutput=0.0  ICPrevInput=0.0  DoSatur=off
  cfblk4 : Product
  cfblk5 : ComplexToRealImag
  cfblk6 : simulink/Math Operations/MinMax Running Resettable  Function=min  vinit=0.0
  cfblk7 : Math  Operator=mod
  cfblk8 : DotProduct  OutDataTypeStr=Inherit: Inherit via internal rule
  cfblk9 : Constant  Value=[-493132407.410047]  SampleTime=1
  cfblk2 : Outport
  wires:
  cfblk6/1 -> cfblk14/1(cfblk1), cfblk25/1
  cfblk12/1(cfblk2) -> cfblk16/1
  cfblk4/1 -> cfblk2/1
  cfblk15/1(cfblk2) -> cfblk12/1(cfblk1)
  cfblk11/1(cfblk2) -> cfblk13/1(cfblk1), cfblk13/3(cfblk8), cfblk19/1, cfblk27/1
  cfblk12/2(cfblk16) -> cfblk14/3(cfblk11)
  cfblk10/1 -> cfblk12/2(cfblk12), cfblk18/4(cfblk12), cfblk17/2(cfblk10), cfblk18/5(cfblk13), cfblk18/7(cfblk15)
  cfblk14/1(cfblk2) -> cfblk7/1
  cfblk15/2(cfblk15) -> cfblk18/2(cfblk10), cfblk13/2(cfblk7)
  cfblk17/1(cfblk2) -> cfblk3/1
  cfblk14/2(cfblk12) -> cfblk8/1
  cfblk13/1(cfblk2) -> cfblk6/1
  cfblk14/3(cfblk13) -> cfblk23/1, cfblk24/1
  cfblk1/1 -> cfblk15/3(cfblk14)
  cfblk5/2 -> cfblk7/2
  cfblk3/1 -> cfblk11/1(cfblk1), cfblk8/2
  cfblk8/1 -> cfblk5/1
  cfblk9/1 -> cfblk4/1, cfblk12/5(cfblk15), cfblk18/6(cfblk14)
  cfblk17/2(cfblk13) -> cfblk18/3(cfblk11)
  cfblk17/3(cfblk14) -> cfblk4/2, cfblk28/1
  cfblk18/2(cfblk17) -> cfblk6/2, cfblk26/1
  cfblk16/1 -> cfblk17/Action
  cfblk16/2 -> cfblk18/Action
  cfblk19/1 -> cfblk18/1(cfblk1)
  cfblk18/1(cfblk2) -> cfblk20/1
  cfblk20/1 -> cfblk17/1(cfblk1)
  cfblk7/1 -> cfblk21/1
  cfblk21/1 -> cfblk14/2(cfblk10)
  cfblk5/1 -> cfblk22/1
  cfblk22/1 -> cfblk15/1(cfblk1)
  cfblk23/1 -> cfblk15/2(cfblk13)
  cfblk24/1 -> cfblk17/4(cfblk12)
  cfblk25/1 -> cfblk12/4(cfblk14)
  cfblk26/1 -> cfblk17/3(cfblk11)
  cfblk27/1 -> cfblk18/8(cfblk16)
  cfblk28/1 -> cfblk12/3(cfblk13)

== system sampleModel653/cfblk191 ==
  cfblk1 : Inport
  Action Port : ActionPort  ActionPortLabel=if(u1 >= 0)
  cfblk10 : Subsystem
  cfblk{11..17} (7 alike) : Delay
  cfblk3 : Sqrt  Operator=rSqrt  AlgorithmType=Newton-Raphson
  cfblk4 : Product
  cfblk5 : Constant  Value=[-587373351.102396]  SampleTime=1
  cfblk6 : Subsystem
  cfblk7 : Subsystem
  cfblk8 : Subsystem
  cfblk9 : Subsystem
  cfblk2 : Outport
  wires:
  cfblk10/2(cfblk15) -> cfblk8/1(cfblk1)
  cfblk4/1 -> cfblk9/3(cfblk12), cfblk6/5(cfblk13)
  cfblk5/1 -> cfblk8/2(cfblk10), cfblk2/1, cfblk7/4(cfblk9)
  cfblk10/3(cfblk16) -> cfblk7/1(cfblk1), cfblk17/1
  cfblk7/3(cfblk12) -> cfblk15/1, cfblk16/1
  cfblk9/1(cfblk2) -> cfblk10/2(cfblk13), cfblk6/3(cfblk11), cfblk7/5(cfblk10), cfblk6/6(cfblk14)
  cfblk6/1(cfblk2) -> cfblk7/2(cfblk7)
  cfblk3/1 -> cfblk6/2(cfblk10), cfblk6/4(cfblk12)
  cfblk8/1(cfblk2) -> cfblk3/1, cfblk12/1
  cfblk1/1 -> cfblk4/1, cfblk8/3(cfblk11), cfblk7/3(cfblk8)
  cfblk10/1(cfblk2) -> cfblk11/1
  cfblk11/1 -> cfblk9/1(cfblk1)
  cfblk12/1 -> cfblk10/3(cfblk14)
  cfblk7/1(cfblk2) -> cfblk13/1
  cfblk13/1 -> cfblk9/2(cfblk11)
  cfblk7/2(cfblk11) -> cfblk14/1
  cfblk14/1 -> cfblk10/1(cfblk1)
  cfblk15/1 -> cfblk6/1(cfblk1)
  cfblk16/1 -> cfblk6/7(cfblk15)
  cfblk17/1 -> cfblk4/2

== system sampleModel653/cfblk192 ==
  cfblk1 : Inport
  cfblk14 : Inport  Port=2
  Action Port : ActionPort  ActionPortLabel=else
  cfblk10 : Product
  cfblk11 : simulink/Math Operations/Slider Gain  gain=1  low=0  high=2
  cfblk12 : UnaryMinus
  cfblk13 : Subsystem
  cfblk18 : Delay
  cfblk19 : Delay
  cfblk20 : Delay
  cfblk3 : DiscreteTransferFcn
  cfblk4 : DiscreteTransferFcn
  cfblk5 : Sin  TimeSource=Use external signal  SampleTime=0
  cfblk6 : Sum  Inputs=+
  cfblk7 : Rounding
  cfblk8 : Squeeze
  cfblk9 : Product  Inputs=**
  cfblk2 : Outport
  cfblk15 : Outport  Port=2
  cfblk16 : Outport  Port=3
  cfblk17 : Outport  Port=4
  wires:
  cfblk13/1(cfblk2) -> cfblk16/1
  cfblk5/1 -> cfblk15/1, cfblk13/1(cfblk1)
  cfblk9/1 -> cfblk8/1
  cfblk7/1 -> cfblk4/1
  cfblk6/1 -> cfblk7/1, cfblk13/4(cfblk14), cfblk13/5(cfblk15)
  cfblk13/2(cfblk16) -> cfblk10/1
  cfblk1/1 -> cfblk17/1, cfblk5/1, cfblk13/2(cfblk12)
  cfblk8/1 -> cfblk11/1
  cfblk14/1 -> cfblk9/1
  cfblk10/1 -> cfblk12/1, cfblk19/1
  cfblk12/1 -> cfblk9/2
  cfblk3/1 -> cfblk2/1, cfblk6/1
  cfblk11/1 -> cfblk18/1
  cfblk18/1 -> cfblk10/2
  cfblk19/1 -> cfblk13/3(cfblk13)
  cfblk4/1 -> cfblk20/1
  cfblk20/1 -> cfblk3/1

== system sampleModel653/cfblk193 ==
  cfblk1 : Inport
  Action Port : ActionPort  ActionPortLabel=if(u1 >= 0)
  cfblk3 : UnitDelay  SampleTime=-1  HasFrameUpgradeWarning=on
  cfblk4 : Math  Operator=log
  cfblk5 : Gain  Gain=[-980019294.842574]
  cfblk6 : simulink/Math Operations/MinMax Running Resettable  Function=min  vinit=0.0
  cfblk7 : Constant  Value=[505936146.843536]  SampleTime=1
  cfblk8 : Constant  Value=[-764117279.732350]  SampleTime=1
  cfblk9 : Subsystem
  cfblk2 : Outport
  wires:
  cfblk8/1 -> cfblk4/1
  cfblk5/1 -> cfblk3/1
  cfblk1/1 -> cfblk9/1(cfblk1)
  cfblk9/1(cfblk2) -> cfblk6/1
  cfblk3/1 -> cfblk6/2
  cfblk7/1 -> cfblk2/1
  cfblk4/1 -> cfblk5/1

== system sampleModel653/cfblk194 ==
  cfblk1 : Inport
  cfblk12 : Inport  Port=2
  Action Port : ActionPort  ActionPortLabel=else
  cfblk10 : Subsystem
  cfblk11 : Subsystem
  cfblk14 : Delay
  cfblk15 : Delay
  cfblk3 : DiscreteFilter
  cfblk4 : Trigonometry
  cfblk5 : PermuteDimensions
  cfblk6 : DotProduct  OutDataTypeStr=Inherit: Inherit via internal rule
  cfblk7 : simulink/Math Operations/Slider Gain  gain=1  low=0  high=2
  cfblk8 : ComplexToMagnitudeAngle
  cfblk9 : Constant  Value=[-870075644.280917]  SampleTime=1
  cfblk2 : Outport
  cfblk13 : Outport  Port=2
  wires:
  cfblk10/1(cfblk2) -> cfblk8/1
  cfblk8/1 -> cfblk7/1
  cfblk7/1 -> cfblk3/1, cfblk11/6(cfblk15)
  cfblk4/1 -> cfblk11/1(cfblk1)
  cfblk10/2(cfblk17) -> cfblk6/1
  cfblk8/2 -> cfblk4/1
  cfblk9/1 -> cfblk2/1, cfblk11/4(cfblk13)
  cfblk12/1 -> cfblk6/2, cfblk11/5(cfblk14), cfblk10/5(cfblk16)
  cfblk3/1 -> cfblk5/1
  cfblk11/1(cfblk2) -> cfblk13/1
  cfblk6/1 -> cfblk11/2(cfblk11)
  cfblk1/1 -> cfblk10/1(cfblk1), cfblk10/4(cfblk15)
  cfblk5/1 -> cfblk11/3(cfblk12)
  cfblk11/2(cfblk16) -> cfblk14/1
  cfblk14/1 -> cfblk10/2(cfblk13)
  cfblk11/3(cfblk17) -> cfblk15/1
  cfblk15/1 -> cfblk10/3(cfblk14)

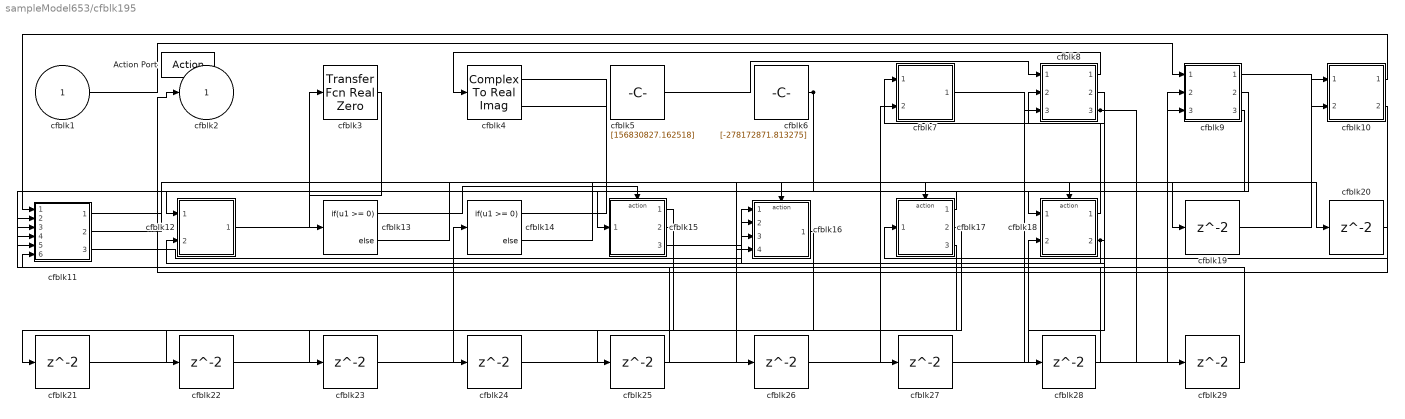
== system sampleModel653/cfblk195 ==
  cfblk1 : Inport
  Action Port : ActionPort  ActionPortLabel=if(u1 >= 0)
  cfblk10 : Subsystem
  cfblk11 : Subsystem
  cfblk12 : Subsystem
  cfblk13 : If  IfExpression=u1 >= 0  SampleTime=1
  cfblk14 : If  IfExpression=u1 >= 0  SampleTime=1
  cfblk15 : Subsystem  TreatAsAtomicUnit=on
  cfblk16 : Subsystem  TreatAsAtomicUnit=on
  cfblk17 : Subsystem  TreatAsAtomicUnit=on
  cfblk18 : Subsystem  TreatAsAtomicUnit=on
  cfblk{19..29} (11 alike) : Delay
  cfblk3 : simulink/Discrete/Transfer Fcn Real Zero  ZeroZ=0.75  ICPrevInput=0.0  DoSatur=off
  cfblk4 : ComplexToRealImag
  cfblk5 : Constant  Value=[156830827.162518]  SampleTime=1
  cfblk6 : Constant  Value=[-278172871.813275]  SampleTime=1
  cfblk7 : Subsystem
  cfblk8 : Subsystem
  cfblk9 : Subsystem
  cfblk2 : Outport
  wires:
  cfblk17/1(cfblk2) -> cfblk12/1(cfblk1)
  cfblk6/1 -> cfblk15/1(cfblk1), cfblk16/4(cfblk17)
  cfblk5/1 -> cfblk8/1(cfblk1)
  cfblk18/1(cfblk2) -> cfblk7/1(cfblk1)
  cfblk8/1(cfblk2) -> cfblk4/1
  cfblk8/2(cfblk6) -> cfblk12/2(cfblk9)
  cfblk1/1 -> cfblk9/1(cfblk1)
  cfblk12/1(cfblk2) -> cfblk3/1
  cfblk15/3(cfblk12) -> cfblk16/1(cfblk1)
  cfblk3/1 -> cfblk13/1
  cfblk18/2(cfblk17) -> cfblk8/2(cfblk4), cfblk16/3(cfblk16)
  cfblk10/1(cfblk2) -> cfblk11/1(cfblk1)
  cfblk10/2(cfblk8) -> cfblk2/1
  cfblk9/1(cfblk2) -> cfblk10/2(cfblk7)
  cfblk11/2(cfblk10) -> cfblk18/1(cfblk1)
  cfblk9/2(cfblk15) -> cfblk11/2(cfblk5)
  cfblk11/3(cfblk11) -> cfblk16/2(cfblk15)
  cfblk8/3(cfblk7) -> cfblk28/1, cfblk29/1
  cfblk9/3(cfblk16) -> cfblk11/5(cfblk8)
  cfblk13/1 -> cfblk15/Action
  cfblk13/2 -> cfblk16/Action
  cfblk14/1 -> cfblk17/Action
  cfblk14/2 -> cfblk18/Action
  cfblk11/1(cfblk2) -> cfblk19/1
  cfblk19/1 -> cfblk10/1(cfblk1)
  cfblk7/1(cfblk2) -> cfblk20/1
  cfblk20/1 -> cfblk17/1(cfblk1)
  cfblk15/1(cfblk2) -> cfblk21/1
  cfblk21/1 -> cfblk7/2(cfblk12)
  cfblk15/2(cfblk11) -> cfblk22/1
  cfblk22/1 -> cfblk9/2(cfblk13)
  cfblk16/1(cfblk2) -> cfblk23/1
  cfblk23/1 -> cfblk14/1
  cfblk17/2(cfblk11) -> cfblk24/1
  cfblk24/1 -> cfblk18/2(cfblk16)
  cfblk17/3(cfblk12) -> cfblk25/1
  cfblk25/1 -> cfblk11/3(cfblk6)
  cfblk4/1 -> cfblk26/1
  cfblk26/1 -> cfblk9/3(cfblk14)
  cfblk4/2 -> cfblk27/1
  cfblk27/1 -> cfblk8/3(cfblk5)
  cfblk28/1 -> cfblk11/4(cfblk7)
  cfblk29/1 -> cfblk11/6(cfblk9)

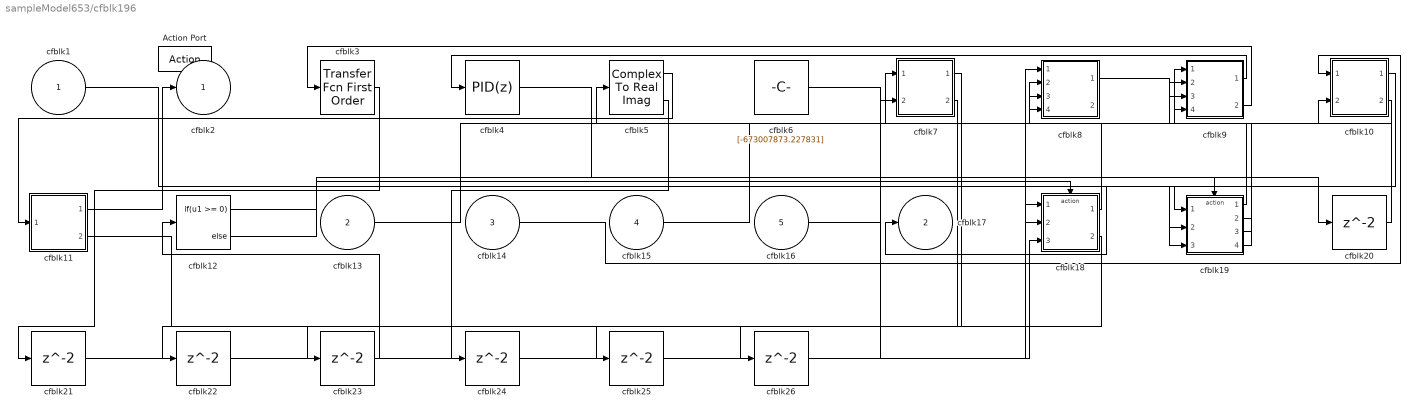
== system sampleModel653/cfblk196 ==
  cfblk1 : Inport
  cfblk13 : Inport  Port=2
  cfblk14 : Inport  Port=3
  cfblk15 : Inport  Port=4
  cfblk16 : Inport  Port=5
  Action Port : ActionPort  ActionPortLabel=else
  cfblk10 : Subsystem
  cfblk11 : Subsystem
  cfblk12 : If  IfExpression=u1 >= 0  SampleTime=1
  cfblk18 : Subsystem  TreatAsAtomicUnit=on
  cfblk19 : Subsystem  TreatAsAtomicUnit=on
  cfblk{20..26} (7 alike) : Delay
  cfblk3 : simulink/Discrete/Transfer Fcn First Order  PoleZ=0.95  ICPrevOutput=0.0  DoSatur=off
  cfblk4 : slpidlib/PID Controller  Controller=PID  Form=Parallel  TimeDomain=Discrete-time  UseExternalTs=off  SampleTime=-1  IntegratorMethod=Forward Euler  FilterMethod=Forward Euler  ControllerParametersSource=internal  P=1  I=1  UseKiTs=off  D=0  N=100  UseFilter=on  TunerSelectOption=Transfer Function Based (PID Tuner App)  InitialConditionSource=internal  InitialConditionForIntegrator=0  InitialConditionForFilter=0  DifferentiatorICPrevScaledInput=0  ExternalReset=none  TrackingMode=off  Kt=1  LimitOutput=off  SatLimitsSource=internal  UpperSaturationLimit=inf  LowerSaturationLimit=-inf  LinearizeAsGain=off  AntiWindupMode=none  Kb=1  LimitIntegrator=off  UpperIntegratorSaturationLimit=inf  LowerIntegratorSaturationLimit=-inf  POutMin=[]  POutMax=[]  IOutMin=[]  IOutMax=[]  DOutMin=[]  DOutMax=[]  NOutMin=[]  NOutMax=[]  SumOutMin=[]  SumOutMax=[]  SaturationOutMin=[]  SaturationOutMax=[]  PParamMin=[]  PParamMax=[]  IParamMin=[]  IParamMax=[]  DParamMin=[]  DParamMax=[]  NParamMin=[]  NParamMax=[]  KbParamMin=[]  KbParamMax=[]  KtParamMin=[]  KtParamMax=[]  KbOutMin=[]  KbOutMax=[]  KtOutMin=[]  KtOutMax=[]  IntegratorOutMin=[]  IntegratorOutMax=[]  FilterOutMin=[]  FilterOutMax=[]  SumI1OutMin=[]  SumI1OutMax=[]  SumI2OutMin=[]  SumI2OutMax=[]  SumI3OutMin=[]  SumI3OutMax=[]  SumI4OutMin=[]  SumI4OutMax=[]  SumDOutMin=[]  SumDOutMax=[]  DifferentiatorOutMin=[]  DifferentiatorOutMax=[]  FilterDiffOutCoefMin=[]  FilterDiffOutCoefMax=[]  ReciprocalOutMin=[]  ReciprocalOutMax=[]  SumDenOutMin=[]  SumDenOutMax=[]  SumNumOutMin=[]  SumNumOutMax=[]  DivideOutMin=[]  DivideOutMax=[]  UdiffTsProdOutMin=[]  UdiffTsProdOutMax=[]  NTsProdOutMin=[]  NTsProdOutMax=[]  UintegralTsProdOutMin=[]  UintegralTsProdOutMax=[]  UngainTsProdOutMin=[]  UngainTsProdOutMax=[]  ClampingZeroOutDataTypeStr=Inherit: Inherit via back propagation  ClampingZeroOutMin=[]  ClampingZeroOutMax=[]  FilterDenConstantOutDataTypeStr=Inherit: Inherit via back propagation  FilterDenConstantOutMin=[]  FilterDenConstantOutMax=[]  PCopyOutDataTypeStr=Inherit: Inherit via back propagation  PCopyOutMin=[]  PCopyOutMax=[]  NCopyOutDataTypeStr=Inherit: Inherit via back propagation  NCopyOutMin=[]  NCopyOutMax=[]  IntegratorContinuousStateAttributes=''  IntegratorStateMustResolveToSignalObject=off  IntegratorRTWStateStorageClass=Auto  FilterContinuousStateAttributes=''  FilterStateMustResolveToSignalObject=off  FilterRTWStateStorageClass=Auto  ParallelPVariant=InternalParameters  IdealPVariant=Disabled  IVariant=InternalParameters  DVariant=InternalParameters  IntegratorVariant=Discrete  SatVariant=Disabled  AWVariant=Passthrough  PCopyVariant=Disabled  TRVariant=Disabled  FdbkBlocksVariant=Forward  IdealPFdbkVariant=Disabled  SatFdbkVariant=Disabled  DerivativeFilterVariant=ForwardEulerFilter  NVariant=InternalParameters  NCopyVariant=Disabled  FilterICVariant=InternalICsFilter  IntegratorICVariant=InternalICs  ExternalResetVariant=Disabled  TRSumVariant=Passthrough  SumFdbkVariant=Disabled  SumVariant=Sum_PID  TsampFilterVariant=InternalTs  TsampNgainVariant=Passthrough  TsampIntegralVariant=Disabled_SignalSpec  ExternalSaturationOutDataTypeStr=Inherit: Same as second input
      settings: LibrarySourceBlock=simulink/Discrete/Discrete PID Controller
  cfblk5 : ComplexToRealImag
  cfblk6 : Constant  Value=[-673007873.227831]  SampleTime=1
  cfblk7 : Subsystem
  cfblk8 : Subsystem
  cfblk9 : Subsystem
  cfblk2 : Outport
  cfblk17 : Outport  Port=2
  wires:
  cfblk13/1 -> cfblk9/1(cfblk1)
  cfblk9/1(cfblk2) -> cfblk4/1
  cfblk5/1 -> cfblk11/1(cfblk1)
  cfblk10/1(cfblk2) -> cfblk17/1
  cfblk11/1(cfblk2) -> cfblk2/1
  cfblk14/1 -> cfblk10/1(cfblk1)
  cfblk18/1(cfblk2) -> cfblk5/1
  cfblk16/1 -> cfblk19/1(cfblk1)
  cfblk15/1 -> cfblk10/2(cfblk10)
  cfblk1/1 -> cfblk19/2(cfblk10)
  cfblk19/1(cfblk2) -> cfblk8/2(cfblk12)
  cfblk19/2(cfblk12) -> cfblk7/1(cfblk1)
  cfblk9/2(cfblk13) -> cfblk3/1
  cfblk10/2(cfblk11) -> cfblk8/3(cfblk13)
  cfblk19/3(cfblk13) -> cfblk8/4(cfblk14)
  cfblk6/1 -> cfblk19/3(cfblk11)
  cfblk8/1(cfblk2) -> cfblk9/3(cfblk11)
  cfblk19/4(cfblk14) -> cfblk9/4(cfblk12)
  cfblk12/1 -> cfblk18/Action
  cfblk12/2 -> cfblk19/Action
  cfblk4/1 -> cfblk20/1
  cfblk20/1 -> cfblk9/2(cfblk10)
  cfblk3/1 -> cfblk21/1
  cfblk21/1 -> cfblk8/1(cfblk1)
  cfblk7/1(cfblk2) -> cfblk22/1
  cfblk22/1 -> cfblk18/1(cfblk1)
  cfblk11/2(cfblk12) -> cfblk23/1
  cfblk23/1 -> cfblk12/1
  cfblk5/2 -> cfblk24/1
  cfblk24/1 -> cfblk18/3(cfblk10)
  cfblk18/2(cfblk11) -> cfblk25/1
  cfblk25/1 -> cfblk7/2(cfblk8)
  cfblk7/2(cfblk9) -> cfblk26/1
  cfblk26/1 -> cfblk18/2(cfblk9)
